simulink model "Assignment_1_3K04"  (R2020a)
settings: Solver=FixedStepAuto  StartTime=0.0  StopTime=10.0  FixedStep=1e-3  RelTol=1e-3  EnableMultiTasking=on
undefined symbols (not defined in the file): D0, D1, D10, D11, D12, D13, D2, D3, D4, D5, D6, D7, D8, D9, PTA0, PTA1, PTA2, PTB23, PTB9, PTC16, PTC17, PTC2, PTC3, PTC4, PTD0, PTD1, PTD2, PTD3
libraries: frdmk64flib x14
settings Model: ExtModeTrigDuration=5  Creator=Stephen Oh  LastModifiedBy=Stephen Oh
settings OptimizationCC: EnhancedBackFolding=on  PassReuseOutputArgsAs=Individual arguments  ZeroExternalMemoryAtStartup=off  ZeroInternalMemoryAtStartup=off  MaxStackSize=64  OptimizeBlockOrder=speed  DifferentSizesBufferReuse=on  OptimizationCustomize=off  EfficientTunableParamExpr=on
settings DebuggingCC: ParameterTunabilityLossMsg=error
settings HardwareCC: ProdBitPerPointer=32  ProdBitPerSizeT=32  ProdBitPerPtrDiffT=32  ProdLargestAtomicInteger=Long  ProdLargestAtomicFloat=Double  ProdWordSize=32  ProdHWDeviceType=ARM Compatible->ARM Cortex
settings SFSimCC: MATLABDynamicMemAlloc=off
settings RTWCC: SystemTargetFile=ert.tlc  HardwareBoard=NXP FRDM-K64F  TemplateMakefile=ert_default_tmf  Toolchain=GNU Tools for ARM Embedded Processors
settings CodeAppCC: ForceParamTrailComments=on  IgnoreCustomStorageClasses=off  OperatorAnnotations=on  SimulinkDataObjDesc=on  SFDataObjDesc=on  InsertBlockDesc=on

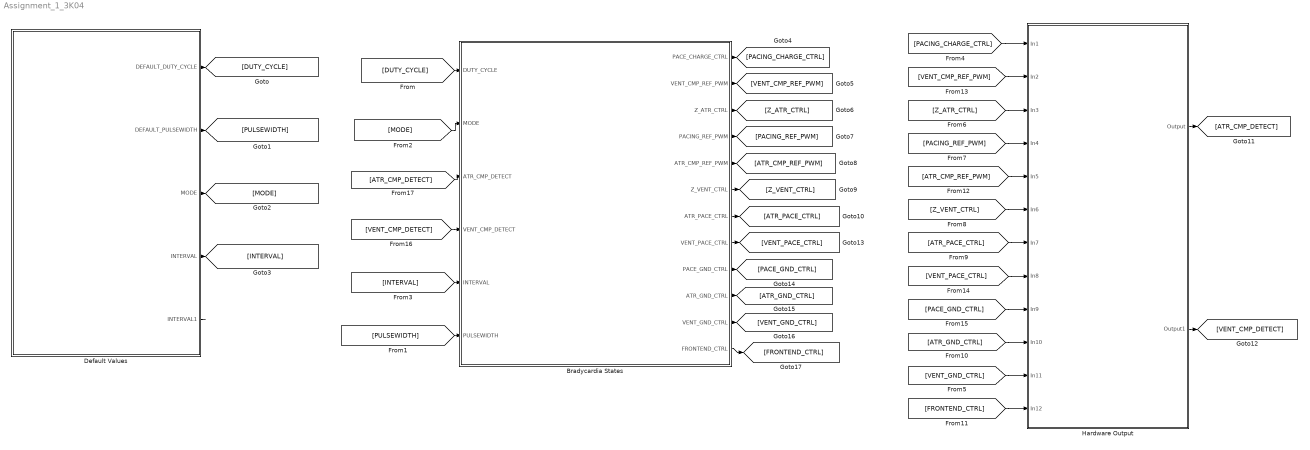
== system Assignment_1_3K04 ==
  Bradycardia States : Stateflow chart  TreatAsAtomicUnit=on
      settings: PortSchema="{\"entries\":[{\"content\":{\"sides\":[{\"content\":{\"connectorIds\":[\"In3\",\"In4\",\"In5\",\"In6\",\"In1\",\"In2\"]},\"type\":\"ConnectorPlacement.EquallySpacedRectSide\",\"uuid\":\"15e03f69-5c25-4f3e-b3fb-d71978e552f4\"},{\"content\":{\"connectorIds\":[\"Out7\",\"Out12\",\"Out4\",\"Out8\",\"Out10\",\"Out5\",\"Out9\",\"Out3\",\"Out6\",\"Out1\",\"Out2\",\"Out11\"],\"side\":\"RIGHT\"},\"type\":\"ConnectorPlacement.EquallySpacedRectSide\",\"uuid\":\"02171bf1-edb1-4b01-9e56-a8642c556ed6\"},{\"content\":{\"connectorIds\":[],\"side\":\"TOP\"},\"type\":\"ConnectorPlacement.EquallySpacedRectSide\",\"uuid\":\"cc6b5506-3435-4740-9e3f-4dfe15d30bff\"}]},\"type\":\"ConnectorPlacement.EquallySpacedConnector\",\"uuid\":\"0ad55da7-1e65-48d0-a0a4-2620ffa94320\"}],\"packageUris\":[\"http://schema.mathworks.com/mf0/Connector/19700101\"],\"version\":\"1.0\"}"
  Default Values : Subsystem
  Hardware Output : Subsystem
  wires:
  Default Values/1(DEFAULT_DUTY_CYCLE) -> [DUTY_CYCLE]
  Default Values/2(DEFAULT_PULSEWIDTH) -> [PULSEWIDTH]
  [DUTY_CYCLE] -> Bradycardia States/3(DUTY_CYCLE)
  [PULSEWIDTH] -> Bradycardia States/2(PULSEWIDTH)
  [MODE] -> Bradycardia States/4(MODE)
  [INTERVAL] -> Bradycardia States/1(INTERVAL)
  Default Values/3(MODE) -> [MODE]
  Default Values/4(INTERVAL) -> [INTERVAL]
  Default Values/5(INTERVAL1) -> ?
  [ATR_GND_CTRL] -> Hardware Output/10(In10)
  [PACING_REF_PWM] -> Hardware Output/4(In4)
  [Z_VENT_CTRL] -> Hardware Output/6(In6)
  [ATR_PACE_CTRL] -> Hardware Output/7(In7)
  Hardware Output/2(Output1) -> [VENT_CMP_DETECT]
  [PACE_GND_CTRL] -> Hardware Output/9(In9)
  [FRONTEND_CTRL] -> Hardware Output/12(In12)
  [VENT_GND_CTRL] -> Hardware Output/11(In11)
  [Z_ATR_CTRL] -> Hardware Output/3(In3)
  [VENT_PACE_CTRL] -> Hardware Output/8(In8)
  [ATR_CMP_REF_PWM] -> Hardware Output/5(In5)
  [VENT_CMP_REF_PWM] -> Hardware Output/2(In2)
  [PACING_CHARGE_CTRL] -> Hardware Output/1(In1)
  Hardware Output/1(Output) -> [ATR_CMP_DETECT]
  Bradycardia States/7(PACE_CHARGE_CTRL) -> [PACING_CHARGE_CTRL]
  Bradycardia States/4(Z_ATR_CTRL) -> [Z_ATR_CTRL]
  Bradycardia States/11(FRONTEND_CTRL) -> [FRONTEND_CTRL]
  Bradycardia States/2(VENT_GND_CTRL) -> [VENT_GND_CTRL]
  Bradycardia States/1(ATR_GND_CTRL) -> [ATR_GND_CTRL]
  Bradycardia States/6(PACE_GND_CTRL) -> [PACE_GND_CTRL]
  Bradycardia States/3(VENT_PACE_CTRL) -> [VENT_PACE_CTRL]
  Bradycardia States/9(ATR_PACE_CTRL) -> [ATR_PACE_CTRL]
  Bradycardia States/5(Z_VENT_CTRL) -> [Z_VENT_CTRL]
  Bradycardia States/10(ATR_CMP_REF_PWM) -> [ATR_CMP_REF_PWM]
  Bradycardia States/8(PACING_REF_PWM) -> [PACING_REF_PWM]
  Bradycardia States/12(VENT_CMP_REF_PWM) -> [VENT_CMP_REF_PWM]
  [ATR_CMP_DETECT] -> Bradycardia States/5(ATR_CMP_DETECT)
  [VENT_CMP_DETECT] -> Bradycardia States/6(VENT_CMP_DETECT)

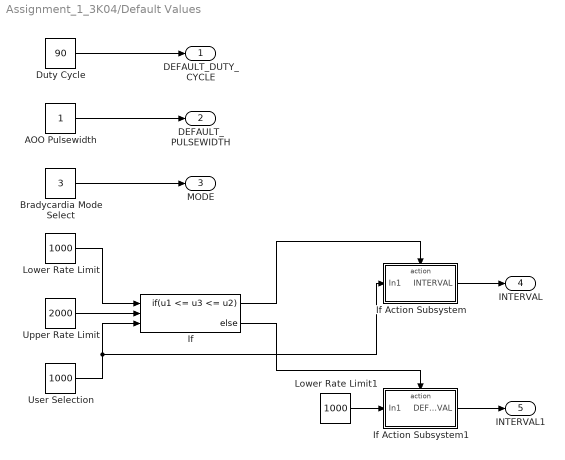
== system Assignment_1_3K04/Default Values ==
  AOO Pulsewidth : Constant
  Bradycardia Mode Select : Constant  Value=3
  Duty Cycle : Constant  Value=90
  If : If  NumInputs=3  IfExpression=u1 <= u3 <= u2
  If Action Subsystem : Subsystem  TreatAsAtomicUnit=on
  If Action Subsystem1 : Subsystem  TreatAsAtomicUnit=on
  Lower Rate Limit : Constant  Value=1000
  Lower Rate Limit1 : Constant  Value=1000
  Upper Rate Limit : Constant  Value=2000
  User Selection : Constant  Value=1000
  DEFAULT_DUTY_CYCLE : Outport
  DEFAULT_PULSEWIDTH : Outport  Port=2
  MODE : Outport  Port=3
  INTERVAL : Outport  Port=4
  INTERVAL1 : Outport  Port=5
  wires:
  Duty Cycle/1 -> DEFAULT_DUTY_CYCLE/1
  AOO Pulsewidth/1 -> DEFAULT_PULSEWIDTH/1
  Lower Rate Limit/1 -> If/1
  Upper Rate Limit/1 -> If/2
  Bradycardia Mode Select/1 -> MODE/1
  User Selection/1 -> If Action Subsystem/1(In1), If/3
  If/1 -> If Action Subsystem/Action
  If Action Subsystem/1(INTERVAL) -> INTERVAL/1
  If/2 -> If Action Subsystem1/Action
  Lower Rate Limit1/1 -> If Action Subsystem1/1(In1)
  If Action Subsystem1/1(DEFAULT INTERVAL) -> INTERVAL1/1

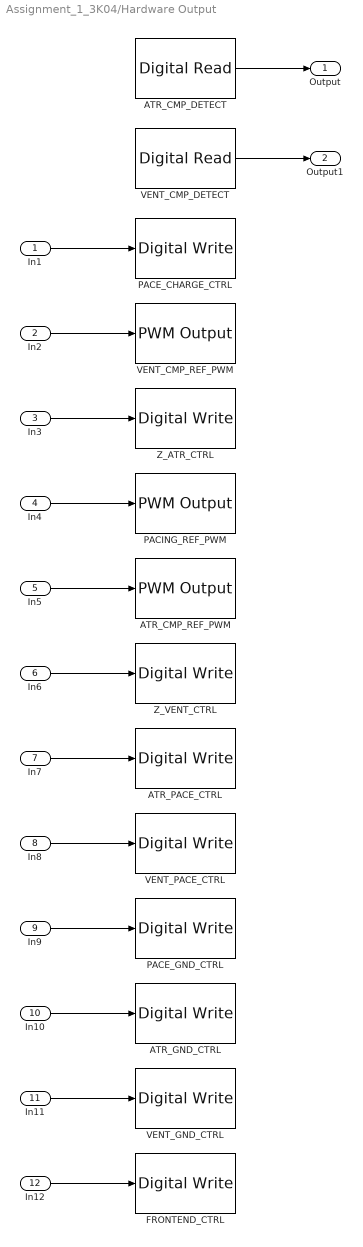
== system Assignment_1_3K04/Hardware Output ==
  In1 : Inport
  In2 : Inport  Port=2
  In3 : Inport  Port=3
  In4 : Inport  Port=4
  In5 : Inport  Port=5
  In6 : Inport  Port=6
  In7 : Inport  Port=7
  In8 : Inport  Port=8
  In9 : Inport  Port=9
  In10 : Inport  Port=10
  In11 : Inport  Port=11
  In12 : Inport  Port=12
  ATR_CMP_DETECT : frdmk64flib/Digital Read  Whichpin=PTC16 (D0)  SampleTime=-1
  ATR_CMP_REF_PWM : frdmk64flib/PWM Output  Whichpin=PTC2 (D6)  InitialFrequency=2000  InitialDutyCycle=30
  ATR_GND_CTRL : frdmk64flib/Digital Write  Whichpin=PTD2 (D11)
  ATR_PACE_CTRL : frdmk64flib/Digital Write  Whichpin=PTA0 (D8)
  FRONTEND_CTRL : frdmk64flib/Digital Write  Whichpin=PTD1 (D13)
  PACE_CHARGE_CTRL : frdmk64flib/Digital Write  Whichpin=PTB9 (D2)
  PACE_GND_CTRL : frdmk64flib/Digital Write  Whichpin=PTD0 (D10)
  PACING_REF_PWM : frdmk64flib/PWM Output  Whichpin=PTA2 (D5)  InitialFrequency=2000  InitialDutyCycle=30
  VENT_CMP_DETECT : frdmk64flib/Digital Read  Whichpin=PTC17 (D1)  SampleTime=-1
  VENT_CMP_REF_PWM : frdmk64flib/PWM Output  Whichpin=PTA1 (D3)  InitialFrequency=2000  InitialDutyCycle=30
  VENT_GND_CTRL : frdmk64flib/Digital Write  Whichpin=PTD3 (D12)
  VENT_PACE_CTRL : frdmk64flib/Digital Write  Whichpin=PTC4 (D9)
  Z_ATR_CTRL : frdmk64flib/Digital Write  Whichpin=PTB23 (D4)
  Z_VENT_CTRL : frdmk64flib/Digital Write  Whichpin=PTC3 (D7)
  Output : Outport
  Output1 : Outport  Port=2
  wires:
  In1/1 -> PACE_CHARGE_CTRL/1
  ATR_CMP_DETECT/1 -> Output/1
  VENT_CMP_DETECT/1 -> Output1/1
  In2/1 -> VENT_CMP_REF_PWM/1
  In3/1 -> Z_ATR_CTRL/1
  In4/1 -> PACING_REF_PWM/1
  In5/1 -> ATR_CMP_REF_PWM/1
  In6/1 -> Z_VENT_CTRL/1
  In7/1 -> ATR_PACE_CTRL/1
  In8/1 -> VENT_PACE_CTRL/1
  In9/1 -> PACE_GND_CTRL/1
  In10/1 -> ATR_GND_CTRL/1
  In11/1 -> VENT_GND_CTRL/1
  In12/1 -> FRONTEND_CTRL/1

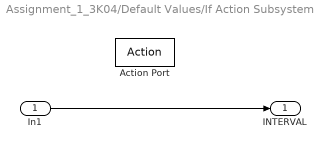
== system Assignment_1_3K04/Default Values/If Action Subsystem ==
  In1 : Inport
  Action Port : ActionPort  ActionPortLabel=if(u1 <= u3 <= u2)
  INTERVAL : Outport
  wires:
  In1/1 -> INTERVAL/1

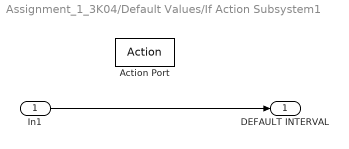
== system Assignment_1_3K04/Default Values/If Action Subsystem1 ==
  In1 : Inport
  Action Port : ActionPort  ActionPortLabel=else
  DEFAULT INTERVAL : Outport
  wires:
  In1/1 -> DEFAULT INTERVAL/1

== stateflow chart Assignment_1_3K04/Bradycardia States ==
  state AOO [group]
    state Charging
      entry:
      %Charging capacitor C22
      %
      ATR_PACE_CTRL = LOW
      VENT_PACE_CTRL = LOW
      PACING_REF_PWM = DUTY_CYCLE
      PACE_CHARGE_CTRL = HIGH
      %Charge release of capacitor C21 into Atrium ground
      PACE_GND_CTRL = HIGH
      VENT_PACE_CTRL = LOW
      Z_ATR_CTRL = LOW
      Z_VENT_CTRL = LOW
      ATR_PACE_CTRL = LOW
      ATR_GND_CTRL = HIGH
      VENT_GND_CTRL = LOW
    state Discharging
      entry:
      %Charge release of capacitor C22 to charge capacitor C21
      %
      PACE_CHARGE_CTRL = LOW
      PACE_GND_CTRL = HIGH
      VENT_PACE_CTRL = LOW
      VENT_GND_CTRL = LOW
      Z_VENT_CTRL = LOW
      Z_ATR_CTRL = LOW
      ATR_GND_CTRL = LOW
      ATR_PACE_CTRL = HIGH
    AOO.Charging -> AOO.Discharging : after(INTERVAL, msec)
    AOO.Discharging -> AOO.Charging : after(PULSEWIDTH, msec)
  state Select
  state VOO [group]
    state Charging
      entry:
      %Charging capacitor C22
      %
      ATR_PACE_CTRL = LOW
      VENT_PACE_CTRL = LOW
      PACING_REF_PWM = DUTY_CYCLE
      PACE_CHARGE_CTRL = HIGH
      %Charge release of capacitor C21 into Atrium ground
      PACE_GND_CTRL = HIGH
      VENT_PACE_CTRL = LOW
      Z_ATR_CTRL = LOW
      Z_VENT_CTRL = LOW
      ATR_PACE_CTRL = LOW
      ATR_GND_CTRL = LOW
      VENT_GND_CTRL = HIGH
    state Discharging
      entry:
      %Charge release of capacitor C22 to charge capacitor C21
      %
      PACE_CHARGE_CTRL = LOW
      PACE_GND_CTRL = HIGH
      ATR_PACE_CTRL = LOW
      ATR_GND_CTRL = LOW
      Z_VENT_CTRL = LOW
      Z_ATR_CTRL = LOW
      VENT_GND_CTRL = LOW
      VENT_PACE_CTRL = HIGH
    VOO.Charging -> VOO.Discharging : after(INTERVAL, msec)
    VOO.Discharging -> VOO.Charging : after(PULSEWIDTH, msec)
  state AAI [group]
    state Test
    state Discharging
      entry:
      %Charge release of capacitor C22 to charge capacitor C21
      %
      PACE_CHARGE_CTRL = LOW
      PACE_GND_CTRL = HIGH
      VENT_PACE_CTRL = LOW
      VENT_GND_CTRL = LOW
      Z_VENT_CTRL = LOW
      Z_ATR_CTRL = LOW
      ATR_GND_CTRL = LOW
      ATR_PACE_CTRL = HIGH
    state Charging
      entry:
      FRONTEND_CTRL = HIGH
      ATR_CMP_REF_PWM = 90
      %Charging capacitor C22
      %
      ATR_PACE_CTRL = LOW
      VENT_PACE_CTRL = LOW
      PACING_REF_PWM = DUTY_CYCLE
      PACE_CHARGE_CTRL = HIGH
      %Charge release of capacitor C21 into Atrium ground
      PACE_GND_CTRL = HIGH
      VENT_PACE_CTRL = LOW
      Z_ATR_CTRL = LOW
      Z_VENT_CTRL = LOW
      ATR_PACE_CTRL = LOW
      ATR_GND_CTRL = HIGH
      VENT_GND_CTRL = LOW
    AAI.Test -> AAI.Charging [order 2] : [ATR_CMP_DETECT == HIGH]
    AAI.Test -> AAI.Discharging [order 1] : after(750, msec)
    AAI.Charging -> AAI.Test : after(250,msec)
    AAI.Discharging -> AAI.Charging : after(PULSEWIDTH, msec)
  state VVI [group]
    state Test
    state Charging
      entry:
      FRONTEND_CTRL = HIGH
      VENT_CMP_REF_PWM = 90
      %Charging capacitor C22
      %
      ATR_PACE_CTRL = LOW
      VENT_PACE_CTRL = LOW
      PACING_REF_PWM = DUTY_CYCLE
      PACE_CHARGE_CTRL = HIGH
      %Charge release of capacitor C21 into Atrium ground
      PACE_GND_CTRL = HIGH
      VENT_PACE_CTRL = LOW
      Z_ATR_CTRL = LOW
      Z_VENT_CTRL = LOW
      ATR_PACE_CTRL = LOW
      ATR_GND_CTRL = LOW
      VENT_GND_CTRL = HIGH
    state Discharging
      entry:
      %Charge release of capacitor C22 to charge capacitor C21
      %
      PACE_CHARGE_CTRL = LOW
      PACE_GND_CTRL = HIGH
      ATR_PACE_CTRL = LOW
      ATR_GND_CTRL = LOW
      Z_VENT_CTRL = LOW
      Z_ATR_CTRL = LOW
      VENT_GND_CTRL = LOW
      VENT_PACE_CTRL = HIGH
    VVI.Test -> VVI.Discharging [order 1] : after(750, msec)
    VVI.Test -> VVI.Charging [order 2] : [VENT_CMP_DETECT == HIGH]
    VVI.Charging -> VVI.Test : after(250,msec)
    VVI.Discharging -> VVI.Charging : after(PULSEWIDTH, msec)
  (default) -> Select
  Select -> AOO.Charging [order 1] : [MODE == 0]
  Select -> VOO.Charging [order 2] : [MODE == 1]
  Select -> VVI.Charging [order 4] : [MODE == 3]
  Select -> AAI.Charging [order 3] : [MODE == 2]
  data: ATR_GND_CTRL output; VENT_GND_CTRL output; VENT_PACE_CTRL output; Z_ATR_CTRL output; Z_VENT_CTRL output; PACE_GND_CTRL output; PACE_CHARGE_CTRL output; PACING_REF_PWM output; ATR_PACE_CTRL output; INTERVAL input; PULSEWIDTH input; DUTY_CYCLE input; HIGH local boolean =true; LOW local boolean =false; MODE input; ATR_CMP_REF_PWM output; FRONTEND_CTRL output; VENT_CMP_REF_PWM output; ATR_CMP_DETECT input; VENT_CMP_DETECT input
